simulink model "mpcpmsm"  (R2019b)
settings: Solver=ode4  StartTime=0.0  StopTime=5  FixedStep=1e-5  RelTol=1e-3
values from neighbouring files (symbols this model uses):
  B = 0.0004924    [PMSM_parameters.m]
  J = 0.0027    [PMSM_parameters.m]
  Ls = 0.000395    [PMSM_parameters.m]
  p = 4    [PMSM_parameters.m]
  Rs = 0.485    [PMSM_parameters.m]
  Sm = 0.1194    [PMSM_parameters.m]
libraries: simulink x2, eeTransforms x1
settings Model: Creator=Windows10  LastModifiedBy=akhil
settings DebuggingCC: UnderSpecifiedDimensionMsg=warning

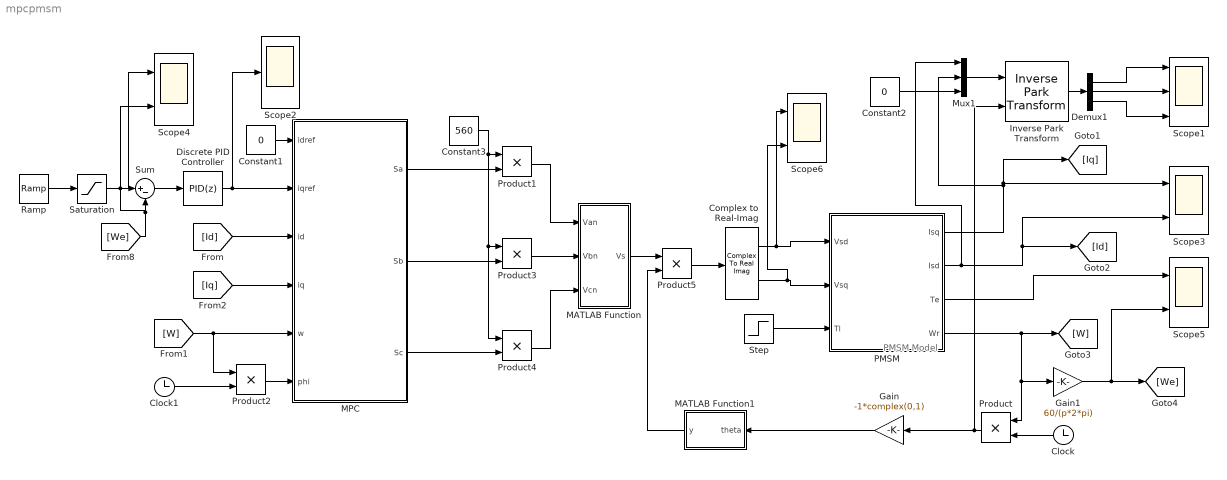
== system mpcpmsm ==
  note: PMSM Model
  Clock : Clock
  Clock1 : Clock
  Complex to Real-Imag : ComplexToRealImag
  Constant1 : Constant  Value=0
  Constant2 : Constant  Value=0
  Constant3 : Constant  Value=560
  Demux1 : Demux  Outputs=3
  Discrete PID Controller : simulink/Continuous/PID Controller  Controller=PID  Form=Parallel  TimeDomain=Discrete-time  SampleTime=-1  IntegratorMethod=Forward Euler  FilterMethod=Forward Euler  ControllerParametersSource=internal  P=0.5  I=1  D=0  UseFilter=on  N=100  TunerSelectOption=Transfer Function Based (PID Tuner App)  InitialConditionSource=internal  InitialConditionForIntegrator=0  InitialConditionForFilter=0  DifferentiatorICPrevScaledInput=0  ExternalReset=none  TrackingMode=off  Kt=1  LimitOutput=on  UpperSaturationLimit=90  LowerSaturationLimit=-90  LinearizeAsGain=on  AntiWindupMode=clamping  Kb=1  POutMin=[]  POutMax=[]  IOutMin=[]  IOutMax=[]  DOutMin=[]  DOutMax=[]  NOutMin=[]  NOutMax=[]  SumOutMin=[]  SumOutMax=[]  SaturationOutMin=[]  SaturationOutMax=[]  PParamMin=[]  PParamMax=[]  IParamMin=[]  IParamMax=[]  DParamMin=[]  DParamMax=[]  NParamMin=[]  NParamMax=[]  KbParamMin=[]  KbParamMax=[]  KtParamMin=[]  KtParamMax=[]  KbOutMin=[]  KbOutMax=[]  KtOutMin=[]  KtOutMax=[]  IntegratorOutMin=[]  IntegratorOutMax=[]  FilterOutMin=[]  FilterOutMax=[]  SumI1OutMin=[]  SumI1OutMax=[]  SumI2OutMin=[]  SumI2OutMax=[]  SumI3OutMin=[]  SumI3OutMax=[]  SumI4OutMin=[]  SumI4OutMax=[]  SumDOutMin=[]  SumDOutMax=[]  DifferentiatorOutMin=[]  DifferentiatorOutMax=[]  FilterDiffOutCoefMin=[]  FilterDiffOutCoefMax=[]  ReciprocalOutMin=[]  ReciprocalOutMax=[]  SumDenOutMin=[]  SumDenOutMax=[]  SumNumOutMin=[]  SumNumOutMax=[]  DivideOutMin=[]  DivideOutMax=[]  IntegratorContinuousStateAttributes=''  IntegratorStateMustResolveToSignalObject=off  IntegratorRTWStateStorageClass=Auto  FilterContinuousStateAttributes=''  FilterStateMustResolveToSignalObject=off  FilterRTWStateStorageClass=Auto  ParallelPVariant=InternalParameters  IdealPVariant=Disabled  IVariant=InternalParameters  DVariant=InternalParameters  IntegratorVariant=Discrete  SatVariant=Enabled  AWVariant=DiscClampingParallel  PCopyVariant=Disabled  TRVariant=Disabled  FdbkBlocksVariant=Forward  IdealPFdbkVariant=Disabled  SatFdbkVariant=Disabled  DerivativeFilterVariant=ForwardEulerFilter  NVariant=InternalParameters  NCopyVariant=Disabled  FilterICVariant=InternalICsFilter  IntegratorICVariant=InternalICs  ExternalResetVariant=Disabled  TRSumVariant=Passthrough  SumFdbkVariant=Disabled  SumVariant=Sum_PID
  Gain : Gain  Gain=-1*complex(0,1)
  Gain1 : Gain  Gain=60/(p*2*pi)
  Inverse Park Transform : eeTransforms/Inverse Park Transform  AxisAlignment=Q-axis  PowerInvariant=off
      settings: SourceProductName=Simscape Electrical
  MATLAB Function : MATLAB Function  TreatAsAtomicUnit=on
  MATLAB Function1 : MATLAB Function  TreatAsAtomicUnit=on
  MPC : MATLAB Function  TreatAsAtomicUnit=on
  Mux1 : Mux  Inputs=3
  PMSM : Subsystem
  Product{,1..5} (6 alike) : Product
  Ramp : simulink/Sources/Ramp  slope=500  start=0  InitialOutput=0
  Saturation : Saturate  UpperLimit=800  LowerLimit=0
  Scope1 : Scope  NumInputPorts=3
  Scope2 : Scope
  Scope{3..6} (4 alike) : Scope  NumInputPorts=2
  Step : Step  Time=2.5  After=10  SampleTime=0
  Sum : Sum  Inputs=|+-
  wires:
  Clock/1 -> Product/2
  PMSM/1(Isq) -> Mux1/2, Scope3/1, [Iq]
  PMSM/4(Wr) -> Gain1/1, Product/1, [W]
  Clock1/1 -> Product2/2
  Product2/1 -> MPC/6(phi)
  PMSM/2(Isd) -> Scope3/2, [Id], Mux1/1
  [Iq] -> MPC/4(iq)
  Constant1/1 -> MPC/1(idref)
  [Id] -> MPC/3(id)
  [W] -> Product2/1, MPC/5(w)
  Sum/1 -> Discrete PID Controller/1
  Gain1/1 -> Scope5/2, [We]
  Ramp/1 -> Saturation/1
  PMSM/3(Te) -> Scope5/1
  Product/1 -> Gain/1, Inverse Park Transform/2
  Mux1/1 -> Inverse Park Transform/1
  Constant2/1 -> Mux1/3
  Inverse Park Transform/1 -> Demux1/1
  Demux1/1 -> Scope1/1
  Demux1/2 -> Scope1/2
  Demux1/3 -> Scope1/3
  MPC/3(Sc) -> Product4/2
  MPC/2(Sb) -> Product3/2
  MPC/1(Sa) -> Product1/2
  Constant3/1 -> Product4/1, Product3/1, Product1/1
  Product1/1 -> MATLAB Function/1(Van)
  Product3/1 -> MATLAB Function/2(Vbn)
  Product4/1 -> MATLAB Function/3(Vcn)
  Product5/1 -> Complex to Real-Imag/1
  MATLAB Function/1(Vs) -> Product5/1
  MATLAB Function1/1(y) -> Product5/2
  Complex to Real-Imag/2 -> Scope6/2, PMSM/2(Vsq)
  Gain/1 -> MATLAB Function1/1(theta)
  Step/1 -> PMSM/3(Tl)
  Discrete PID Controller/1 -> MPC/2(iqref), Scope2/1
  [We] -> Scope4/2, Sum/2
  Saturation/1 -> Scope4/1, Sum/1
  Complex to Real-Imag/1 -> Scope6/1, PMSM/1(Vsd)

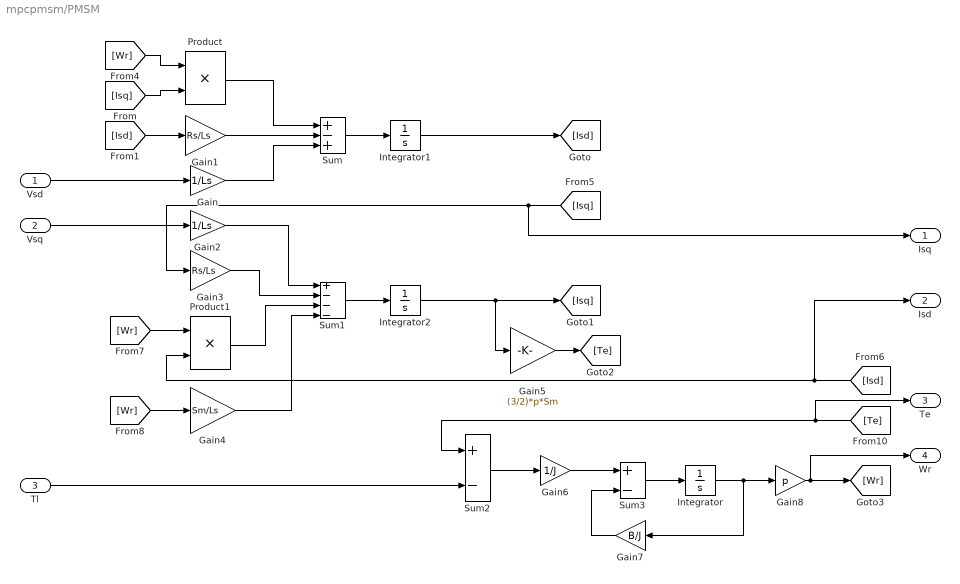
== system mpcpmsm/PMSM ==
  Vsd : Inport
  Vsq : Inport  Port=2
  Tl : Inport  Port=3
  Gain : Gain  Gain=1/Ls
  Gain1 : Gain  Gain=Rs/Ls
  Gain2 : Gain  Gain=1/Ls
  Gain3 : Gain  Gain=Rs/Ls
  Gain4 : Gain  Gain=Sm/Ls
  Gain5 : Gain  Gain=(3/2)*p*Sm
  Gain6 : Gain  Gain=1/J
  Gain7 : Gain  Gain=B/J
  Gain8 : Gain  Gain=p
  Integrator : Integrator
  Integrator1 : Integrator
  Integrator2 : Integrator
  Product : Product
  Product1 : Product
  Sum : Sum  Inputs=+-+
  Sum1 : Sum  Inputs=+---
  Sum2 : Sum  Inputs=+-
  Sum3 : Sum  Inputs=+-
  Isq : Outport
  Isd : Outport  Port=2
  Te : Outport  Port=3
  Wr : Outport  Port=4
  wires:
  Gain5/1 -> [Te]
  [Wr] -> Gain4/1
  [Isq] -> Isq/1, Gain3/1
  [Te] -> Te/1, Sum2/1
  Integrator2/1 -> Gain5/1, [Isq]
  Gain6/1 -> Sum3/1
  Sum1/1 -> Integrator2/1
  Gain/1 -> Sum/3
  Integrator/1 -> Gain8/1, Gain7/1
  Tl/1 -> Sum2/2
  Gain8/1 -> Wr/1, [Wr]
  Gain2/1 -> Sum1/1
  Sum3/1 -> Integrator/1
  Vsd/1 -> Gain/1
  Sum2/1 -> Gain6/1
  [Isd] -> Isd/1, Product1/2
  Gain7/1 -> Sum3/2
  Gain3/1 -> Sum1/2
  Gain4/1 -> Sum1/4
  [Wr] -> Product/1
  Integrator1/1 -> [Isd]
  [Isq] -> Product/2
  Product1/1 -> Sum1/3
  [Wr] -> Product1/1
  Product/1 -> Sum/1
  Gain1/1 -> Sum/2
  [Isd] -> Gain1/1
  Sum/1 -> Integrator1/1
  Vsq/1 -> Gain2/1

== matlab function mpcpmsm/MATLAB Function ==
  data: Van input; Vs output; Vbn input; Vcn input
function Vs = fcn(Van,Vbn,Vcn)

a=complex(cos(2*pi/3),sin(2*pi/3)); 
Vs =(2/3)*(Van+(a*Vbn)+((a^2)*Vcn)) ;

== matlab function mpcpmsm/MATLAB Function1 ==
  data: theta input; y output
function y = fcn(theta)

y = exp((theta));

== matlab function mpcpmsm/MPC ==
  settings: updateMethod=DISCRETE
  data: idref input; Sa output; iqref input; id input; iq input; w input; Sb output; Sc output; phi input
function [Sa, Sb, Sc] = mpc(idref, iqref, id, iq, w,phi) 
%% Initialisation 
R = 0.485;
Ls = 0.000395;
Vdc = 560;
Lambda_f = 0.1194;
Ts = 1e-5;
imax=80;
p=4;
cost=1e14; 
persistent state_1; 
if isempty(state_1) 
    state_1 = 1; 
end

    %% Switching functions 
    S = [0 0 0; 1 0 0; 1 1 0; 0 1 0; 0 1 1; 0 0 1; 1 0 1; 1 1 1]; 
    
    for i=1:8
    %% Voltage applied k+1  
    ud = Vdc*(2/3)*(S(i,1)*cos(phi) + S(i,2)*cos(phi-2*pi/3) + S(i,3)*cos(phi + 2*pi/3)); 
    uq = Vdc*(2/3)* (-S(i,1) *sin(phi) - S(i,2)*sin(phi- 2*pi/3) - S(i,3)*sin(phi + 2*pi/3));
    %% Motor Model (Estimated current vector for k+1) 
    id1 = ((1 -(R*Ts)/Ls)*id) + ((Ts*ud)/Ls) + (w*Ts*iq) ; 
    iq1 = ((1 - (R*Ts)/Ls)*iq) + ((Ts*uq)/Ls) - ((w*Ts*id)) - (((w*Ts*Lambda_f)/Ls)); 
 
%      %% Motor Model (Predicted current values for k+2) 
%      idp2 = ((1 - (R*Ts)/Ls)*id1) + ((Ts*ud)/Ls) + ((w*Ls*Ts*iq1)/Ls) ; 
%      iqp2 = ((1 -(R*Ts)/Ls)*iq1) + ((Ts*uq)/Ls) - ((w*Ls*Ts*id1)/Ls) - ((w*Ts*Lambda_f)/Ls);

     % Hard constraints
     f = 0; 
    if abs(id1) > imax || abs(iq1) > imax 
           f = 1e14; 
    end
      current_cost=(idref-id1)^2 + (iqref-iq1)^2 +f; 
% current_cost= abs(idref-id1) + abs(iqref-iq1);
     if(current_cost<cost) 
     state_1=i;
     cost=current_cost;
     end
      
   end
   Sa = S(state_1,1);
   Sb = S(state_1,2); 
   Sc = S(state_1,3);
